simulink model "tracking_control"  (Simulink 10.3)
settings: Solver=ode45  StartTime=0.0  StopTime=200  MaxStep=0.02  RelTol=1e-3  EnableMultiTasking=on
libraries: simulink x2
settings Model: Creator=Administrator  LastModifiedBy=1179956468
settings SolverCC: AlgebraicLoopSolver=LineSearch
settings DataIOCC: LimitDataPoints=on
settings DebuggingCC: AlgebraicLoopMsg=none
settings GRTTargetCC: CombineOutputUpdateFcns=on  GRTInterface=off

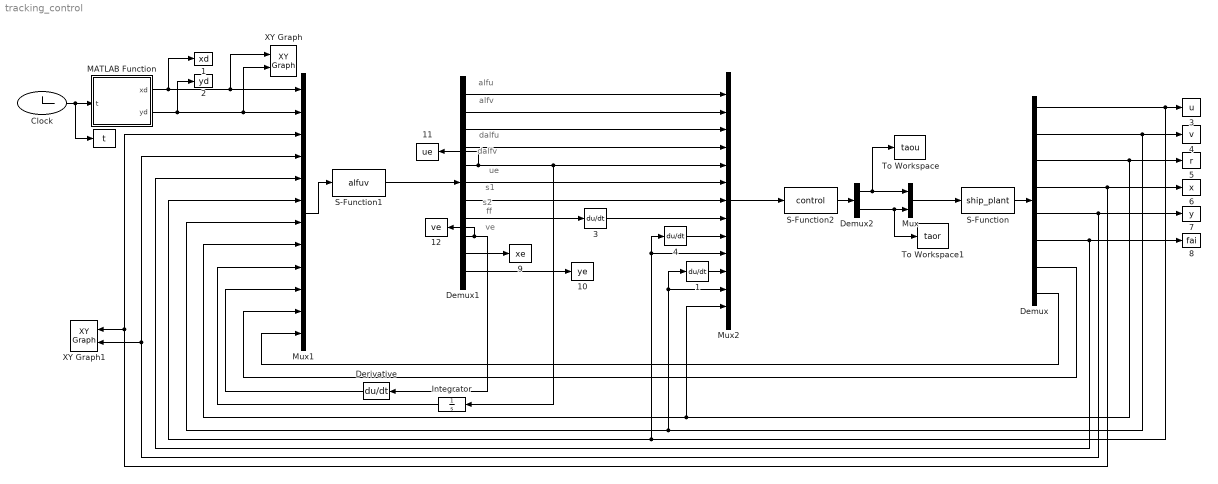
== system tracking_control ==
  note: alfu
  note: alfv
  note: dalfu
  note: dalfv
  note: ue
  note: ve
  note: ff
  note: s1
  note: s2
  " " : ToWorkspace  VariableName=t  SampleTime=-1
  "   1" : Derivative
  "   3" : Derivative
  "   4" : Derivative
  " 1" : ToWorkspace  VariableName=xd  SampleTime=-1
  " 10" : ToWorkspace  VariableName=ye  SampleTime=-1
  " 11" : ToWorkspace  VariableName=ue  SampleTime=-1
  " 12" : ToWorkspace  VariableName=ve  SampleTime=-1
  " 2" : ToWorkspace  VariableName=yd  SampleTime=-1
  " 3" : ToWorkspace  VariableName=u  SampleTime=-1
  " 4" : ToWorkspace  VariableName=v  SampleTime=-1
  " 5" : ToWorkspace  VariableName=r  SampleTime=-1
  " 6" : ToWorkspace  VariableName=x  SampleTime=-1
  " 7" : ToWorkspace  VariableName=y  SampleTime=-1
  " 8" : ToWorkspace  VariableName=fai  SampleTime=-1
  " 9" : ToWorkspace  VariableName=xe  SampleTime=-1
  Clock : Clock
  Demux : Demux  Outputs=8
  Demux1 : Demux  Outputs=11
  Demux2 : Demux  Outputs=2
  Derivative : Derivative
  Integrator : Integrator
  MATLAB Function : MATLAB Function  TreatAsAtomicUnit=on
  Mux : Mux  Inputs=2
  Mux1 : Mux  Inputs=12
  Mux2 : Mux  Inputs=13
  S-Function : S-Function  FunctionName=ship_plant  SFunctionDeploymentMode=off  EnableBusSupport=off
  S-Function1 : S-Function  FunctionName=alfuv  SFunctionDeploymentMode=off  EnableBusSupport=off
  S-Function2 : S-Function  FunctionName=control  SFunctionDeploymentMode=off  EnableBusSupport=off
  To Workspace : ToWorkspace  VariableName=taou  SampleTime=-1
  To Workspace1 : ToWorkspace  VariableName=taor  SampleTime=-1
  XY Graph : simulink/Sinks/XY Graph  xmin=-350  xmax=350  ymin=-350  ymax=350  st=-1
  XY Graph1 : simulink/Sinks/XY Graph  xmin=-350  xmax=350  ymin=-350  ymax=350  st=-1
  wires:
  Clock/1 -> MATLAB Function/1(t), " "/1
  S-Function/1 -> Demux/1
  Demux/1 -> " 3"/1, Mux1/6, "   4"/1, Mux2/10
  Demux/2 -> " 4"/1, Mux1/7, Mux2/12, "   1"/1
  Demux/3 -> " 5"/1, Mux1/8, Mux2/13
  Demux/4 -> " 6"/1, Mux1/3, XY Graph1/1
  Demux/5 -> " 7"/1, Mux1/4, XY Graph1/2
  Demux/6 -> " 8"/1, Mux1/5
  Mux/1 -> S-Function/1
  Mux1/1 -> S-Function1/1
  S-Function1/1 -> Demux1/1
  Demux1/1 -> Mux2/1
  S-Function2/1 -> Demux2/1
  Demux1/2 -> Mux2/2
  Demux1/3 -> Mux2/3
  Demux1/4 -> Mux2/4
  Demux1/5 -> Mux2/5, Integrator/1, " 11"/1
  Mux2/1 -> S-Function2/1
  "   3"/1 -> Mux2/8
  "   4"/1 -> Mux2/9
  "   1"/1 -> Mux2/11
  Demux2/1 -> To Workspace/1, Mux/1
  Demux2/2 -> Mux/2, To Workspace1/1
  MATLAB Function/2(yd) -> " 2"/1, Mux1/2, XY Graph/2
  Derivative/1 -> Mux1/10
  Integrator/1 -> Mux1/9
  Demux/7 -> Mux1/11
  Demux/8 -> Mux1/12
  Demux1/10 -> " 9"/1
  Demux1/11 -> " 10"/1
  Demux1/9 -> Derivative/1, " 12"/1
  Demux1/8 -> "   3"/1
  Demux1/6 -> Mux2/6
  Demux1/7 -> Mux2/7
  MATLAB Function/1(xd) -> " 1"/1, Mux1/1, XY Graph/1

== matlab function MATLAB Function ==
  data: t input double; xd output double; yd output double
function [xd,yd]= fcn(t)
%#codegen
% xd=200*sin(0.02*t);
% yd=200*cos(0.02*t);
% xd=200*sin(0.05*t);
% yd=200*cos(0.05*t);
% xd=200*sin(0.02*t+pi/4);
% yd=200*cos(0.02*t+pi/4);
% xd=300*sin(0.03*t);
% yd=300*cos(0.03*t);
xd=10*t;
yd=1*t;
